simulink model "saturationdynamic_param_test"  (Simulink 8.7)
settings: Solver=ode45  StartTime=0.0  StopTime=10.0  RelTol=1e-3
libraries: simulink x4
settings Model: Creator=arnaud  LastModifiedBy=hamza
settings DataIOCC: SaveFormat=Structure  SignalLoggingSaveFormat=ModelDataLogs
settings OptimizationCC: ExpressionDepthLimit=2147483647
settings DebuggingCC: SolverPrmCheckMsg=warning  FcnCallInpInsideContextMsg=UseLocalSettings  StateNameClashWarn=warning  StrictBusMsg=Warning
settings GRTTargetCC: GeneratePreprocessorConditionals=Use local settings  CombineOutputUpdateFcns=off  GRTInterface=on

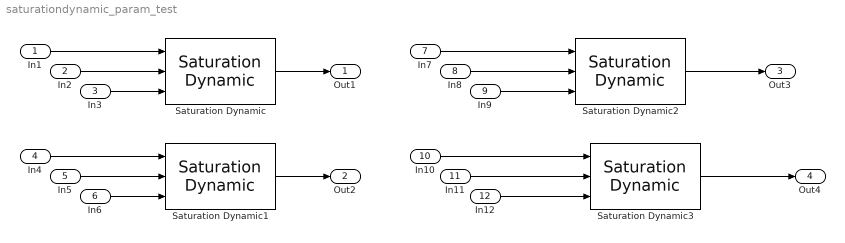
== system saturationdynamic_param_test ==
  In1 : Inport
  In2 : Inport  Port=2
  In3 : Inport  Port=3
  In4 : Inport  Port=4  OutDataTypeStr=int8
  In5 : Inport  Port=5
  In6 : Inport  Port=6  OutDataTypeStr=int8
  In7 : Inport  Port=7  PortDimensions=2
  In8 : Inport  Port=8  PortDimensions=2
  In9 : Inport  Port=9  PortDimensions=2
  In10 : Inport  Port=10  PortDimensions=[2 3]
  In11 : Inport  Port=11  PortDimensions=[2 3]
  In12 : Inport  Port=12  PortDimensions=[2 3]
  Saturation Dynamic{,1..3} (4 alike) : simulink/Discontinuities/Saturation Dynamic  OutMin=[]  OutMax=[]  OutDataTypeStr=Inherit: Same as second input  OutDataType=sfix(16)  OutScaling=2^-10  DoSatur=off
  Out1 : Outport
  Out2 : Outport  Port=2
  Out3 : Outport  Port=3
  Out4 : Outport  Port=4
  wires:
  Saturation Dynamic/1 -> Out1/1
  In1/1 -> Saturation Dynamic/1
  In2/1 -> Saturation Dynamic/2
  In3/1 -> Saturation Dynamic/3
  Saturation Dynamic1/1 -> Out2/1
  In4/1 -> Saturation Dynamic1/1
  In5/1 -> Saturation Dynamic1/2
  In6/1 -> Saturation Dynamic1/3
  Saturation Dynamic2/1 -> Out3/1
  In7/1 -> Saturation Dynamic2/1
  In8/1 -> Saturation Dynamic2/2
  In9/1 -> Saturation Dynamic2/3
  Saturation Dynamic3/1 -> Out4/1
  In10/1 -> Saturation Dynamic3/1
  In11/1 -> Saturation Dynamic3/2
  In12/1 -> Saturation Dynamic3/3
